simulink model "PMSMDrive"  (R2021b)
settings: Solver=VariableStepAuto  StartTime=0.0  StopTime=50e-3  MaxStep=10e-6  RelTol=1e-3
libraries: EMD x3, simulink_extras x1
settings Model: Creator=Szalay  LastModifiedBy=Szalay

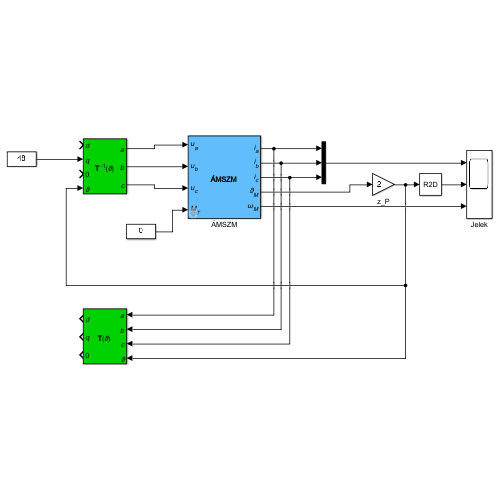
[thumbnail: Simulink's stored preview of the top-level diagram]
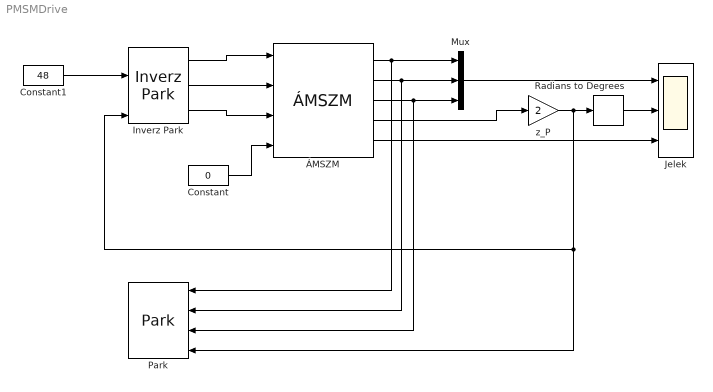
== system PMSMDrive ==
  Constant : Constant  Value=0
  Constant1 : Constant  Value=48
  Inverz Park : EMD/Inverz Park  SystemSampleTime=-1  VariantActivationTime=update diagram  Latency=0  AutoFrameSizeCalculation=off
  Jelek : Scope  NumInputPorts=3
  Mux : Mux  Inputs=3
  Park : EMD/Park  SystemSampleTime=-1  VariantActivationTime=update diagram  Latency=0  AutoFrameSizeCalculation=off
  Radians to Degrees : simulink_extras/Transformations/Radians to Degrees
  z_P : Gain  Gain=2
  ÁMSZM : EMD/ÁMSZM  R=0.5  maskL_d=140  maskL_q=190  maskF_PM=25  z_P=2  maskJ=200  B=1e-5  i_d0=0  i_q0=0  w_M0=0  maskTh_M0=0
  wires:
  ÁMSZM/1 -> Park/1, Mux/1
  ÁMSZM/2 -> Park/2, Mux/2
  ÁMSZM/3 -> Park/3, Mux/3
  Mux/1 -> Jelek/1
  ÁMSZM/4 -> z_P/1
  ÁMSZM/5 -> Jelek/3
  Constant/1 -> ÁMSZM/4
  Radians to Degrees/1 -> Jelek/2
  z_P/1 -> Park/4, Inverz Park/4, Radians to Degrees/1
  Inverz Park/1 -> ÁMSZM/1
  Inverz Park/2 -> ÁMSZM/2
  Inverz Park/3 -> ÁMSZM/3
  Constant1/1 -> Inverz Park/2
